simulink model "Long"  (R2022a)
settings: Solver=ode4  StartTime=0.0  StopTime=100  MaxStep=0.2  RelTol=1e-3
values from neighbouring files (symbols this model uses):
  A_long_full1 = [-0.572980534968 -0.172917573343 0.00419953690196 0 0.0281274513379 -0.574800189634 0.0069673880694 0 -20.2670925764 -184.283117809 -0.503819275398 1 ... (16 elements, 4x4)]    [matlab.mat]
  B_long_full = [Xde                         Xdth ... (first row only)    [Longituidinal.m]    (also in matlab.mat = [1.19  0.00228; -29.7  9.94e-05; -4.7809712  -3.02176e-08; 0)
  C_long_full = eye(4)    [Longituidinal.m]    (also in matlab.mat = [1 0 0 0 0 1 0 0 0 0 1 0 ... (16 elements, 4x4)])
libraries: simulink_extras x3, cstblocks x3, slpidlib x3
settings Model: Creator=Mohamed Ismail  LastModifiedBy=Mohamed Ismail

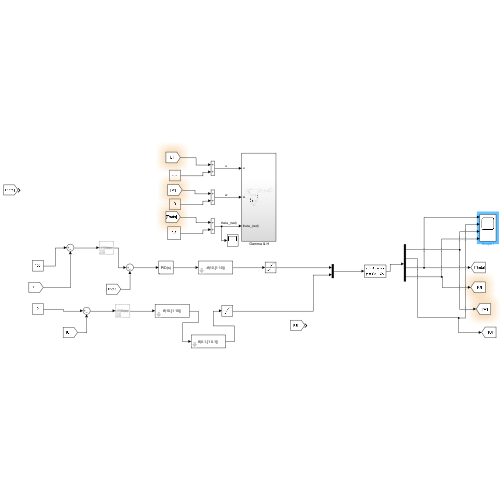
[thumbnail: Simulink's stored preview of the top-level diagram]
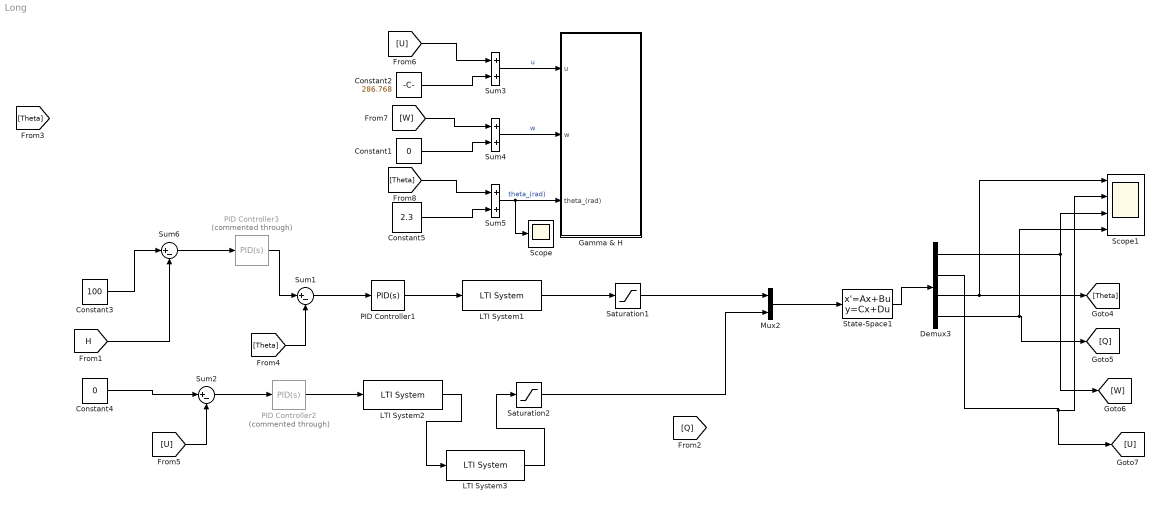
== system Long ==
  " Gamma & H" : Subsystem
  Constant1 : Constant  Value=0
  Constant2 : Constant  Value=286.768
  Constant3 : Constant  Value=100
  Constant4 : Constant  Value=0
  Constant5 : Constant  Value=2.3
  Demux3 : Demux
  LTI System1 : cstblocks/LTI System  sys=-tf(10,[1 10])  IC=[]
  LTI System2 : cstblocks/LTI System  sys=tf(10,[1 10])  IC=[]
  LTI System3 : cstblocks/LTI System  sys=tf(0.1,[1 0.1])  IC=[]
  Mux2 : Mux  Inputs=2
  PID Controller1 : slpidlib/PID Controller  Controller=PID  Form=Parallel  TimeDomain=Continuous-time  UseExternalTs=off  SampleTime=-1  IntegratorMethod=Forward Euler  FilterMethod=Forward Euler  ControllerParametersSource=internal  P=0.390554703212597  I=.00167275571490297  UseKiTs=off  D=12.1787166967996  N=100  UseFilter=on  TunerSelectOption=Transfer Function Based (PID Tuner App)  InitialConditionSource=internal  InitialConditionForIntegrator=0  InitialConditionForFilter=0  DifferentiatorICPrevScaledInput=0  ExternalReset=none  TrackingMode=off  Kt=1  LimitOutput=off  SatLimitsSource=internal  UpperSaturationLimit=inf  LowerSaturationLimit=-inf  LinearizeAsGain=on  AntiWindupMode=none  Kb=1  POutMin=[]  POutMax=[]  IOutMin=[]  IOutMax=[]  DOutMin=[]  DOutMax=[]  NOutMin=[]  NOutMax=[]  SumOutMin=[]  SumOutMax=[]  SaturationOutMin=[]  SaturationOutMax=[]  PParamMin=[]  PParamMax=[]  IParamMin=[]  IParamMax=[]  DParamMin=[]  DParamMax=[]  NParamMin=[]  NParamMax=[]  KbParamMin=[]  KbParamMax=[]  KtParamMin=[]  KtParamMax=[]  KbOutMin=[]  KbOutMax=[]  KtOutMin=[]  KtOutMax=[]  IntegratorOutMin=[]  IntegratorOutMax=[]  FilterOutMin=[]  FilterOutMax=[]  SumI1OutMin=[]  SumI1OutMax=[]  SumI2OutMin=[]  SumI2OutMax=[]  SumI3OutMin=[]  SumI3OutMax=[]  SumI4OutMin=[]  SumI4OutMax=[]  SumDOutMin=[]  SumDOutMax=[]  DifferentiatorOutMin=[]  DifferentiatorOutMax=[]  FilterDiffOutCoefMin=[]  FilterDiffOutCoefMax=[]  ReciprocalOutMin=[]  ReciprocalOutMax=[]  SumDenOutMin=[]  SumDenOutMax=[]  SumNumOutMin=[]  SumNumOutMax=[]  DivideOutMin=[]  DivideOutMax=[]  UdiffTsProdOutMin=[]  UdiffTsProdOutMax=[]  NTsProdOutMin=[]  NTsProdOutMax=[]  UintegralTsProdOutMin=[]  UintegralTsProdOutMax=[]  UngainTsProdOutMin=[]  UngainTsProdOutMax=[]  IntegratorContinuousStateAttributes=''  IntegratorStateMustResolveToSignalObject=off  IntegratorRTWStateStorageClass=Auto  FilterContinuousStateAttributes=''  FilterStateMustResolveToSignalObject=off  FilterRTWStateStorageClass=Auto  ParallelPVariant=InternalParameters  IdealPVariant=Disabled  IVariant=InternalParameters  DVariant=InternalParameters  IntegratorVariant=Continuous  SatVariant=Disabled  AWVariant=Passthrough  PCopyVariant=Disabled  TRVariant=Disabled  FdbkBlocksVariant=Forward  IdealPFdbkVariant=Disabled  SatFdbkVariant=Disabled  DerivativeFilterVariant=ContFilter  NVariant=InternalParameters  NCopyVariant=Disabled  FilterICVariant=InternalICsFilter  IntegratorICVariant=InternalICs  ExternalResetVariant=Disabled  TRSumVariant=Passthrough  SumFdbkVariant=Disabled  SumVariant=Sum_PID  TsampFilterVariant=InternalTs  TsampNgainVariant=Passthrough  TsampIntegralVariant=Passthrough  ExternalSaturationOutDataTypeStr=Inherit: Same as second input  aMode=0
  PID Controller2 : slpidlib/PID Controller  Commented=through  Controller=PID  Form=Parallel  TimeDomain=Continuous-time  UseExternalTs=off  SampleTime=-1  IntegratorMethod=Forward Euler  FilterMethod=Forward Euler  ControllerParametersSource=internal  P=0.390554703212597  I=.00167275571490297  UseKiTs=off  D=12.1787166967996  N=100  UseFilter=on  TunerSelectOption=Transfer Function Based (PID Tuner App)  InitialConditionSource=internal  InitialConditionForIntegrator=0  InitialConditionForFilter=0  DifferentiatorICPrevScaledInput=0  ExternalReset=none  TrackingMode=off  Kt=1  LimitOutput=off  SatLimitsSource=internal  UpperSaturationLimit=inf  LowerSaturationLimit=-inf  LinearizeAsGain=on  AntiWindupMode=none  Kb=1  POutMin=[]  POutMax=[]  IOutMin=[]  IOutMax=[]  DOutMin=[]  DOutMax=[]  NOutMin=[]  NOutMax=[]  SumOutMin=[]  SumOutMax=[]  SaturationOutMin=[]  SaturationOutMax=[]  PParamMin=[]  PParamMax=[]  IParamMin=[]  IParamMax=[]  DParamMin=[]  DParamMax=[]  NParamMin=[]  NParamMax=[]  KbParamMin=[]  KbParamMax=[]  KtParamMin=[]  KtParamMax=[]  KbOutMin=[]  KbOutMax=[]  KtOutMin=[]  KtOutMax=[]  IntegratorOutMin=[]  IntegratorOutMax=[]  FilterOutMin=[]  FilterOutMax=[]  SumI1OutMin=[]  SumI1OutMax=[]  SumI2OutMin=[]  SumI2OutMax=[]  SumI3OutMin=[]  SumI3OutMax=[]  SumI4OutMin=[]  SumI4OutMax=[]  SumDOutMin=[]  SumDOutMax=[]  DifferentiatorOutMin=[]  DifferentiatorOutMax=[]  FilterDiffOutCoefMin=[]  FilterDiffOutCoefMax=[]  ReciprocalOutMin=[]  ReciprocalOutMax=[]  SumDenOutMin=[]  SumDenOutMax=[]  SumNumOutMin=[]  SumNumOutMax=[]  DivideOutMin=[]  DivideOutMax=[]  UdiffTsProdOutMin=[]  UdiffTsProdOutMax=[]  NTsProdOutMin=[]  NTsProdOutMax=[]  UintegralTsProdOutMin=[]  UintegralTsProdOutMax=[]  UngainTsProdOutMin=[]  UngainTsProdOutMax=[]  IntegratorContinuousStateAttributes=''  IntegratorStateMustResolveToSignalObject=off  IntegratorRTWStateStorageClass=Auto  FilterContinuousStateAttributes=''  FilterStateMustResolveToSignalObject=off  FilterRTWStateStorageClass=Auto  ParallelPVariant=InternalParameters  IdealPVariant=Disabled  IVariant=InternalParameters  DVariant=InternalParameters  IntegratorVariant=Continuous  SatVariant=Disabled  AWVariant=Passthrough  PCopyVariant=Disabled  TRVariant=Disabled  FdbkBlocksVariant=Forward  IdealPFdbkVariant=Disabled  SatFdbkVariant=Disabled  DerivativeFilterVariant=ContFilter  NVariant=InternalParameters  NCopyVariant=Disabled  FilterICVariant=InternalICsFilter  IntegratorICVariant=InternalICs  ExternalResetVariant=Disabled  TRSumVariant=Passthrough  SumFdbkVariant=Disabled  SumVariant=Sum_PID  TsampFilterVariant=InternalTs  TsampNgainVariant=Passthrough  TsampIntegralVariant=Passthrough  ExternalSaturationOutDataTypeStr=Inherit: Same as second input  aMode=0
  PID Controller3 : slpidlib/PID Controller  Commented=through  Controller=PID  Form=Parallel  TimeDomain=Continuous-time  UseExternalTs=off  SampleTime=-1  IntegratorMethod=Forward Euler  FilterMethod=Forward Euler  ControllerParametersSource=internal  P=-0.0382128564943725  I=-0.0250605387164027  UseKiTs=off  D=0.00185748677478788  N=11.4609039827728  UseFilter=on  TunerSelectOption=Transfer Function Based (PID Tuner App)  InitialConditionSource=internal  InitialConditionForIntegrator=0  InitialConditionForFilter=0  DifferentiatorICPrevScaledInput=0  ExternalReset=none  TrackingMode=off  Kt=1  LimitOutput=off  SatLimitsSource=internal  UpperSaturationLimit=inf  LowerSaturationLimit=-inf  LinearizeAsGain=on  AntiWindupMode=none  Kb=1  POutMin=[]  POutMax=[]  IOutMin=[]  IOutMax=[]  DOutMin=[]  DOutMax=[]  NOutMin=[]  NOutMax=[]  SumOutMin=[]  SumOutMax=[]  SaturationOutMin=[]  SaturationOutMax=[]  PParamMin=[]  PParamMax=[]  IParamMin=[]  IParamMax=[]  DParamMin=[]  DParamMax=[]  NParamMin=[]  NParamMax=[]  KbParamMin=[]  KbParamMax=[]  KtParamMin=[]  KtParamMax=[]  KbOutMin=[]  KbOutMax=[]  KtOutMin=[]  KtOutMax=[]  IntegratorOutMin=[]  IntegratorOutMax=[]  FilterOutMin=[]  FilterOutMax=[]  SumI1OutMin=[]  SumI1OutMax=[]  SumI2OutMin=[]  SumI2OutMax=[]  SumI3OutMin=[]  SumI3OutMax=[]  SumI4OutMin=[]  SumI4OutMax=[]  SumDOutMin=[]  SumDOutMax=[]  DifferentiatorOutMin=[]  DifferentiatorOutMax=[]  FilterDiffOutCoefMin=[]  FilterDiffOutCoefMax=[]  ReciprocalOutMin=[]  ReciprocalOutMax=[]  SumDenOutMin=[]  SumDenOutMax=[]  SumNumOutMin=[]  SumNumOutMax=[]  DivideOutMin=[]  DivideOutMax=[]  UdiffTsProdOutMin=[]  UdiffTsProdOutMax=[]  NTsProdOutMin=[]  NTsProdOutMax=[]  UintegralTsProdOutMin=[]  UintegralTsProdOutMax=[]  UngainTsProdOutMin=[]  UngainTsProdOutMax=[]  IntegratorContinuousStateAttributes=''  IntegratorStateMustResolveToSignalObject=off  IntegratorRTWStateStorageClass=Auto  FilterContinuousStateAttributes=''  FilterStateMustResolveToSignalObject=off  FilterRTWStateStorageClass=Auto  ParallelPVariant=InternalParameters  IdealPVariant=Disabled  IVariant=InternalParameters  DVariant=InternalParameters  IntegratorVariant=Continuous  SatVariant=Disabled  AWVariant=Passthrough  PCopyVariant=Disabled  TRVariant=Disabled  FdbkBlocksVariant=Forward  IdealPFdbkVariant=Disabled  SatFdbkVariant=Disabled  DerivativeFilterVariant=ContFilter  NVariant=InternalParameters  NCopyVariant=Disabled  FilterICVariant=InternalICsFilter  IntegratorICVariant=InternalICs  ExternalResetVariant=Disabled  TRSumVariant=Passthrough  SumFdbkVariant=Disabled  SumVariant=Sum_PID  TsampFilterVariant=InternalTs  TsampNgainVariant=Passthrough  TsampIntegralVariant=Passthrough  ExternalSaturationOutDataTypeStr=Inherit: Same as second input  aMode=0
  Saturation1 : Saturate  UpperLimit=30*pi/180  LowerLimit=-30*pi/180  ZeroCross=off
  Saturation2 : Saturate  UpperLimit=3700  LowerLimit=-3*3700  ZeroCross=off
  Scope : Scope
  Scope1 : Scope  NumInputPorts=4
  State-Space1 : StateSpace  A=A_long_full1  B=B_long_full  C=C_long_full  D=[0,0;0,0;0,0;0,0;]  InitialCondition=0  ParameterTunability=Unconstrained
  Sum1 : Sum  Inputs=|+-
  Sum2 : Sum  Inputs=|+-
  Sum3 : Sum
  Sum4 : Sum
  Sum5 : Sum
  Sum6 : Sum  Inputs=|+-
  wires:
  Saturation2/1 -> Mux2/2
  LTI System1/1 -> Saturation1/1
  Sum1/1 -> PID Controller1/1
  Saturation1/1 -> Mux2/1
  Demux3/3 -> Scope1/1, [Theta]
  PID Controller1/1 -> LTI System1/1
  Mux2/1 -> State-Space1/1
  State-Space1/1 -> Demux3/1
  PID Controller2/1 -> LTI System2/1
  Demux3/1 -> [W], Scope1/3
  Demux3/2 -> [U], Scope1/2
  Constant4/1 -> Sum2/1
  [Theta] -> Sum1/2
  [U] -> Sum2/2
  Sum2/1 -> PID Controller2/1
  LTI System2/1 -> LTI System3/1
  LTI System3/1 -> Saturation2/1
  Constant5/1 -> Sum5/2
  Constant1/1 -> Sum4/2
  [W] -> Sum4/1
  Sum4/1 -> " Gamma & H"/2(w)  "w"
  Sum5/1 -> Scope/1, " Gamma & H"/3(theta_(rad))  "theta_(rad)"
  Constant2/1 -> Sum3/2
  [Theta] -> Sum5/1
  Sum3/1 -> " Gamma & H"/1(u)  "u"
  [U] -> Sum3/1
  PID Controller3/1 -> Sum1/1
  Sum6/1 -> PID Controller3/1
  Constant3/1 -> Sum6/1
  [H] -> Sum6/2
  Demux3/4 -> Scope1/4, [Q]

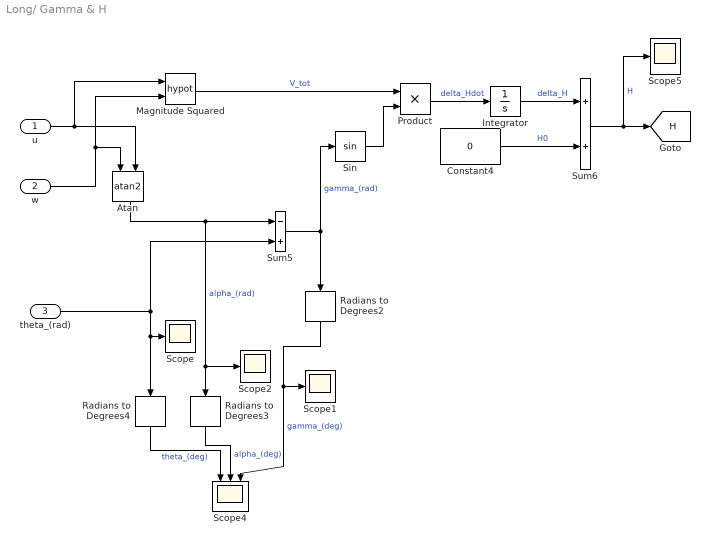
== system Long/ Gamma & H ==
  u : Inport
  w : Inport  Port=2
  theta_(rad) : Inport  Port=3
  Atan : Trigonometry  Operator=atan2
  Constant4 : Constant  Value=0
  Integrator : Integrator
  Magnitude Squared : Math  Operator=hypot  SignedPower=on
  Product : Product
  Radians to Degrees2 : simulink_extras/Transformations/Radians to Degrees
  Radians to Degrees3 : simulink_extras/Transformations/Radians to Degrees
  Radians to Degrees4 : simulink_extras/Transformations/Radians to Degrees
  Scope{,1..2,5} (4 alike) : Scope
  Scope4 : Scope  NumInputPorts=3
  Sin : Trigonometry
  Sum5 : Sum  Inputs=-+
  Sum6 : Sum
  tag scope: H=global
  wires:
  Radians to Degrees3/1 -> Scope4/2  "alpha_(deg)"
  Constant4/1 -> Sum6/2  "H0"
  u/1 -> Magnitude Squared/1, Atan/2
  Magnitude Squared/1 -> Product/1  "V_tot"
  Sin/1 -> Product/2
  Product/1 -> Integrator/1  "delta_Hdot"
  Sum6/1 -> Scope5/1, [H]  "H"
  Radians to Degrees2/1 -> Scope1/1, Scope4/3  "gamma_(deg)"
  Sum5/1 -> Radians to Degrees2/1, Sin/1  "gamma_(rad)"
  theta_(rad)/1 -> Scope/1, Radians to Degrees4/1, Sum5/2
  Integrator/1 -> Sum6/1  "delta_H"
  w/1 -> Magnitude Squared/2, Atan/1
  Radians to Degrees4/1 -> Scope4/1  "theta_(deg)"
  Atan/1 -> Sum5/1, Radians to Degrees3/1, Scope2/1  "alpha_(rad)"
